simulink model "teppo"  (R2019a)
settings: Solver=VariableStepAuto  StartTime=0.0  StopTime=10.0  RelTol=1e-3
libraries: simulink x4, vrlib x2, visionsinks x1
settings Model: Creator=Arjun  LastModifiedBy=Arjun
settings DebuggingCC: UnderSpecifiedDimensionMsg=warning

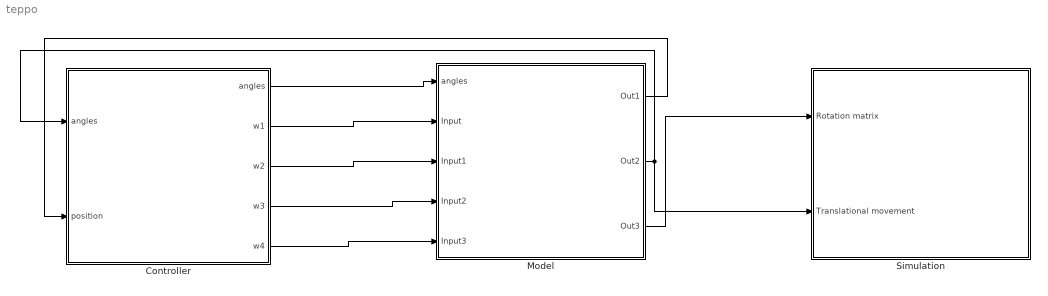
== system teppo ==
  "Controller " : Subsystem
  Model : Subsystem
  Simulation : Subsystem
  wires:
  "Controller "/1("angles ") -> Model/1("angles ")
  Model/3(Out3) -> Simulation/1(Rotation matrix)
  Model/1(Out1) -> "Controller "/2(position)
  Model/2(Out2) -> "Controller "/1(angles), Simulation/2(Translational movement)
  "Controller "/2(w1) -> Model/2(Input)
  "Controller "/3(w2) -> Model/3(Input1)
  "Controller "/4(w3) -> Model/4(Input2)
  "Controller "/5(w4) -> Model/5(Input3)

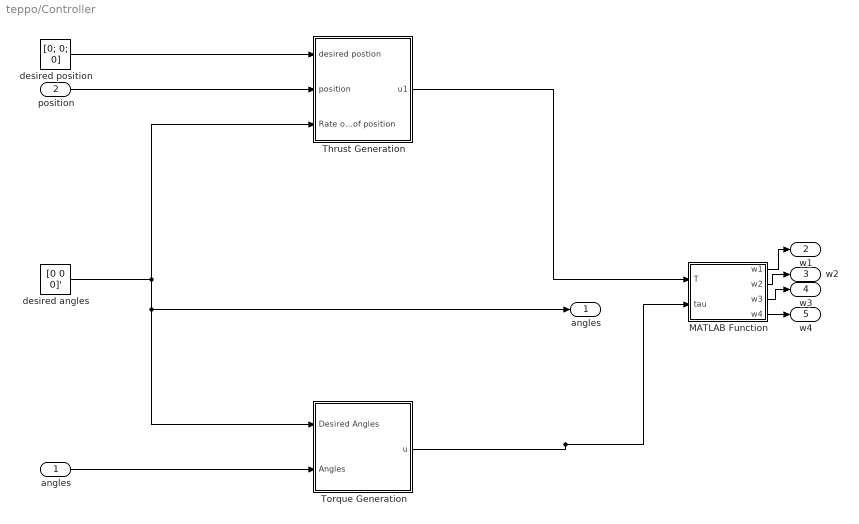
== system teppo/Controller  ==
  angles : Inport
  position : Inport  Port=2
  MATLAB Function : MATLAB Function  TreatAsAtomicUnit=on
  Thrust Generation : Subsystem
  Torque Generation : Subsystem
  desired angles : Constant  Value=[0 0 0]'
  desired position : Constant  Value=[0; 0; 0]
  "angles " : Outport
  w1 : Outport  Port=2
  w2 : Outport  Port=3
  w3 : Outport  Port=4
  w4 : Outport  Port=5
  wires:
  desired angles/1 -> Torque Generation/1("Desired Angles "), "angles "/1, Thrust Generation/3("Rate of change of position ")
  desired position/1 -> Thrust Generation/1("desired postion ")
  position/1 -> Thrust Generation/2(position)
  Thrust Generation/1(u1) -> MATLAB Function/1(T)
  angles/1 -> Torque Generation/2(Angles)
  Torque Generation/1(u) -> MATLAB Function/2(tau)
  MATLAB Function/1(w1) -> w1/1
  MATLAB Function/2(w2) -> w2/1
  MATLAB Function/3(w3) -> w3/1
  MATLAB Function/4(w4) -> w4/1

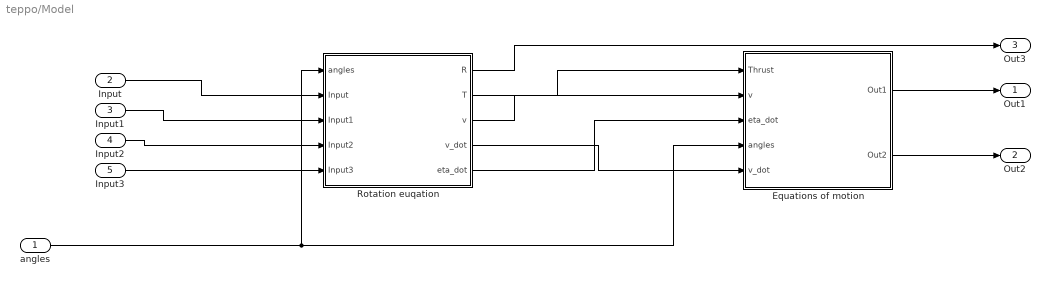
== system teppo/Model ==
  "angles " : Inport
  Input : Inport  Port=2
  Input1 : Inport  Port=3
  Input2 : Inport  Port=4
  Input3 : Inport  Port=5
  Equations of motion : Subsystem
  Rotation euqation : Subsystem
  Out1 : Outport
  Out2 : Outport  Port=2
  Out3 : Outport  Port=3
  wires:
  Rotation euqation/2(T) -> Equations of motion/1(Thrust)
  Rotation euqation/3("v ") -> Equations of motion/2("v ")
  "angles "/1 -> Equations of motion/4("angles "), Rotation euqation/1(angles)
  Rotation euqation/4("v_dot ") -> Equations of motion/5(v_dot)
  Equations of motion/2(Out2) -> Out2/1
  Equations of motion/1(Out1) -> Out1/1
  Rotation euqation/1(R) -> Out3/1
  Input/1 -> Rotation euqation/2(Input)
  Input1/1 -> Rotation euqation/3(Input1)
  Input2/1 -> Rotation euqation/4(Input2)
  Input3/1 -> Rotation euqation/5(Input3)
  Rotation euqation/5(eta_dot) -> Equations of motion/3("eta_dot ")

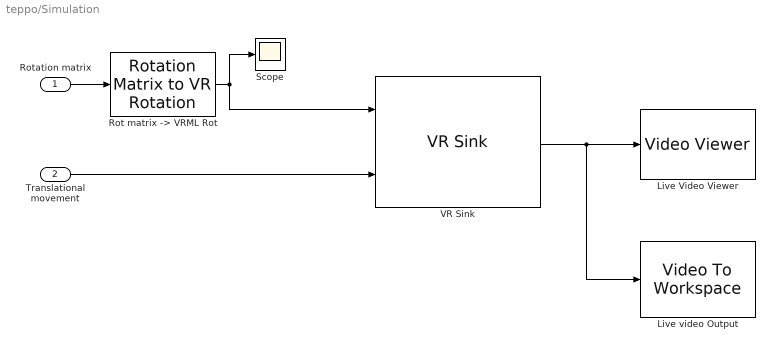
== system teppo/Simulation ==
  Rotation matrix : Inport
  Translational movement : Inport  Port=2
  Live Video Viewer : VideoViewer  FigPos=[1287 1075 375 346]
  Live video Output : visionsinks/Video To Workspace  VariableName=output  NumInputs=1  DataLimit=10  DecimationFactor=1  LogFi=off  InPortLabels=R|G|B
      settings: SourceProductName=Computer Vision Toolbox  SourceProductBaseCode=VP
  "Rot matrix -> VRML Rot" : vrlib/Utilities/Rotation Matrix to VR Rotation  maxzero=0
      settings: SourceProductName=Simulink 3D Animation  SourceProductBaseCode=VR
  Scope : Scope
  VR Sink : vrlib/VR Sink  InstantiateOnLoad=on  SampleTime=0.1  ViewEnable=on  RemoteChange=off  RemoteView=off  FieldsWritten=Quadcopter.rotation.4.1.1.double#Quadcopter.translation.3.1.1.double  WorldFileName=Quadcopter.wrl  AutoView=off  VideoDimensions=[277 277]  AllowVariableSize=off
      settings: SourceProductName=Simulink
  wires:
  "Rot matrix -> VRML Rot"/1 -> VR Sink/1, Scope/1
  Rotation matrix/1 -> "Rot matrix -> VRML Rot"/1
  VR Sink/1 -> Live video Output/1, Live Video Viewer/1
  Translational movement/1 -> VR Sink/2

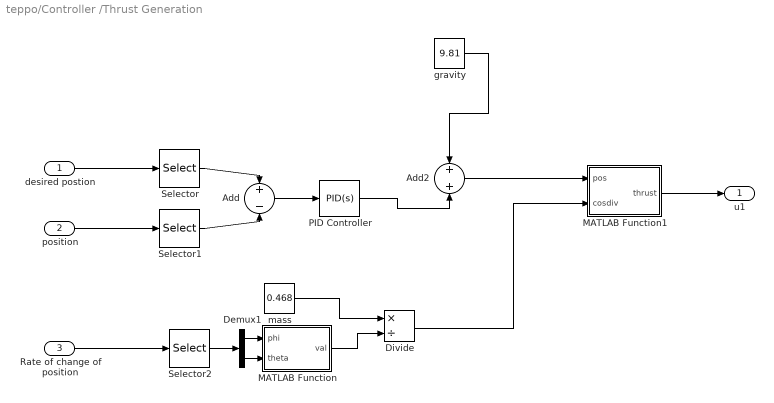
== system teppo/Controller /Thrust Generation ==
  "desired postion " : Inport
  position : Inport  Port=2
  "Rate of change of position " : Inport  Port=3
  Add : Sum  Inputs=+-
  Add2 : Sum
  Demux1 : Demux  Outputs=2
  Divide : Product  Inputs=*/
  MATLAB Function : MATLAB Function  TreatAsAtomicUnit=on
  MATLAB Function1 : MATLAB Function  TreatAsAtomicUnit=on
  PID Controller : simulink/Continuous/PID Controller  Controller=PID  Form=Parallel  TimeDomain=Continuous-time  SampleTime=-1  IntegratorMethod=Forward Euler  FilterMethod=Forward Euler  ControllerParametersSource=internal  P=1.5  I=1  D=2.5  UseFilter=on  N=100  TunerSelectOption=Transfer Function Based (PID Tuner App)  InitialConditionSource=internal  InitialConditionForIntegrator=0  InitialConditionForFilter=0  DifferentiatorICPrevScaledInput=0  ExternalReset=none  TrackingMode=off  Kt=1  LimitOutput=off  UpperSaturationLimit=inf  LowerSaturationLimit=-inf  LinearizeAsGain=on  AntiWindupMode=none  Kb=1  POutMin=[]  POutMax=[]  IOutMin=[]  IOutMax=[]  DOutMin=[]  DOutMax=[]  NOutMin=[]  NOutMax=[]  SumOutMin=[]  SumOutMax=[]  SaturationOutMin=[]  SaturationOutMax=[]  PParamMin=[]  PParamMax=[]  IParamMin=[]  IParamMax=[]  DParamMin=[]  DParamMax=[]  NParamMin=[]  NParamMax=[]  KbParamMin=[]  KbParamMax=[]  KtParamMin=[]  KtParamMax=[]  KbOutMin=[]  KbOutMax=[]  KtOutMin=[]  KtOutMax=[]  IntegratorOutMin=[]  IntegratorOutMax=[]  FilterOutMin=[]  FilterOutMax=[]  SumI1OutMin=[]  SumI1OutMax=[]  SumI2OutMin=[]  SumI2OutMax=[]  SumI3OutMin=[]  SumI3OutMax=[]  SumI4OutMin=[]  SumI4OutMax=[]  SumDOutMin=[]  SumDOutMax=[]  DifferentiatorOutMin=[]  DifferentiatorOutMax=[]  FilterDiffOutCoefMin=[]  FilterDiffOutCoefMax=[]  ReciprocalOutMin=[]  ReciprocalOutMax=[]  SumDenOutMin=[]  SumDenOutMax=[]  SumNumOutMin=[]  SumNumOutMax=[]  DivideOutMin=[]  DivideOutMax=[]  IntegratorContinuousStateAttributes=''  IntegratorStateMustResolveToSignalObject=off  IntegratorRTWStateStorageClass=Auto  FilterContinuousStateAttributes=''  FilterStateMustResolveToSignalObject=off  FilterRTWStateStorageClass=Auto  ParallelPVariant=InternalParameters  IdealPVariant=Disabled  IVariant=InternalParameters  DVariant=InternalParameters  IntegratorVariant=Continuous  SatVariant=Disabled  AWVariant=Passthrough  PCopyVariant=Disabled  TRVariant=Disabled  FdbkBlocksVariant=Forward  IdealPFdbkVariant=Disabled  SatFdbkVariant=Disabled  DerivativeFilterVariant=ContFilter  NVariant=InternalParameters  NCopyVariant=Disabled  FilterICVariant=InternalICsFilter  IntegratorICVariant=InternalICs  ExternalResetVariant=Disabled  TRSumVariant=Passthrough  SumFdbkVariant=Disabled  SumVariant=Sum_PID
  Selector : Selector  InputPortWidth=3  IndexOptions=Index vector (dialog)  Indices=[3]  OutputSizes=1
  Selector1 : Selector  InputPortWidth=3  IndexOptions=Index vector (dialog)  Indices=[3]  OutputSizes=1
  Selector2 : Selector  InputPortWidth=3  IndexOptions=Index vector (dialog)  Indices=[1 2]  OutputSizes=1
  "gravity " : Constant  Value=9.81
  "mass " : Constant  Value=0.468
  u1 : Outport
  wires:
  "mass "/1 -> Divide/1
  "desired postion "/1 -> Selector/1
  Demux1/2 -> MATLAB Function/2(theta)
  Demux1/1 -> MATLAB Function/1(phi)
  Divide/1 -> MATLAB Function1/2(cosdiv)
  Add2/1 -> MATLAB Function1/1(pos)
  MATLAB Function/1(val) -> Divide/2
  Selector2/1 -> Demux1/1
  MATLAB Function1/1(thrust) -> u1/1
  "Rate of change of position "/1 -> Selector2/1
  "gravity "/1 -> Add2/1
  position/1 -> Selector1/1
  Selector/1 -> Add/1
  Selector1/1 -> Add/2
  Add/1 -> PID Controller/1
  PID Controller/1 -> Add2/2

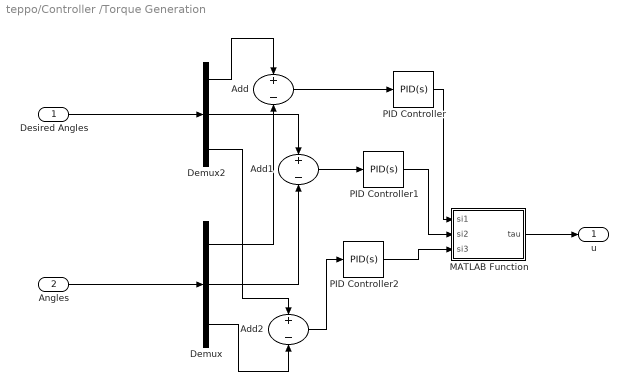
== system teppo/Controller /Torque Generation ==
  "Desired Angles " : Inport
  Angles : Inport  Port=2
  Add : Sum  Inputs=+-
  Add1 : Sum  Inputs=+-
  Add2 : Sum  Inputs=+-
  Demux : Demux  Outputs=3
  Demux2 : Demux  Outputs=3
  MATLAB Function : MATLAB Function  TreatAsAtomicUnit=on
  PID Controller : simulink/Continuous/PID Controller  Controller=PID  Form=Parallel  TimeDomain=Continuous-time  SampleTime=-1  IntegratorMethod=Forward Euler  FilterMethod=Forward Euler  ControllerParametersSource=internal  P=1  I=1  D=0  UseFilter=on  N=100  TunerSelectOption=Transfer Function Based (PID Tuner App)  InitialConditionSource=internal  InitialConditionForIntegrator=0  InitialConditionForFilter=0  DifferentiatorICPrevScaledInput=0  ExternalReset=none  TrackingMode=off  Kt=1  LimitOutput=off  UpperSaturationLimit=inf  LowerSaturationLimit=-inf  LinearizeAsGain=on  AntiWindupMode=none  Kb=1  POutMin=[]  POutMax=[]  IOutMin=[]  IOutMax=[]  DOutMin=[]  DOutMax=[]  NOutMin=[]  NOutMax=[]  SumOutMin=[]  SumOutMax=[]  SaturationOutMin=[]  SaturationOutMax=[]  PParamMin=[]  PParamMax=[]  IParamMin=[]  IParamMax=[]  DParamMin=[]  DParamMax=[]  NParamMin=[]  NParamMax=[]  KbParamMin=[]  KbParamMax=[]  KtParamMin=[]  KtParamMax=[]  KbOutMin=[]  KbOutMax=[]  KtOutMin=[]  KtOutMax=[]  IntegratorOutMin=[]  IntegratorOutMax=[]  FilterOutMin=[]  FilterOutMax=[]  SumI1OutMin=[]  SumI1OutMax=[]  SumI2OutMin=[]  SumI2OutMax=[]  SumI3OutMin=[]  SumI3OutMax=[]  SumI4OutMin=[]  SumI4OutMax=[]  SumDOutMin=[]  SumDOutMax=[]  DifferentiatorOutMin=[]  DifferentiatorOutMax=[]  FilterDiffOutCoefMin=[]  FilterDiffOutCoefMax=[]  ReciprocalOutMin=[]  ReciprocalOutMax=[]  SumDenOutMin=[]  SumDenOutMax=[]  SumNumOutMin=[]  SumNumOutMax=[]  DivideOutMin=[]  DivideOutMax=[]  IntegratorContinuousStateAttributes=''  IntegratorStateMustResolveToSignalObject=off  IntegratorRTWStateStorageClass=Auto  FilterContinuousStateAttributes=''  FilterStateMustResolveToSignalObject=off  FilterRTWStateStorageClass=Auto  ParallelPVariant=InternalParameters  IdealPVariant=Disabled  IVariant=InternalParameters  DVariant=InternalParameters  IntegratorVariant=Continuous  SatVariant=Disabled  AWVariant=Passthrough  PCopyVariant=Disabled  TRVariant=Disabled  FdbkBlocksVariant=Forward  IdealPFdbkVariant=Disabled  SatFdbkVariant=Disabled  DerivativeFilterVariant=ContFilter  NVariant=InternalParameters  NCopyVariant=Disabled  FilterICVariant=InternalICsFilter  IntegratorICVariant=InternalICs  ExternalResetVariant=Disabled  TRSumVariant=Passthrough  SumFdbkVariant=Disabled  SumVariant=Sum_PID
  PID Controller1 : simulink/Continuous/PID Controller  Controller=PID  Form=Parallel  TimeDomain=Continuous-time  SampleTime=-1  IntegratorMethod=Forward Euler  FilterMethod=Forward Euler  ControllerParametersSource=internal  P=1  I=1  D=0  UseFilter=on  N=100  TunerSelectOption=Transfer Function Based (PID Tuner App)  InitialConditionSource=internal  InitialConditionForIntegrator=0  InitialConditionForFilter=0  DifferentiatorICPrevScaledInput=0  ExternalReset=none  TrackingMode=off  Kt=1  LimitOutput=off  UpperSaturationLimit=inf  LowerSaturationLimit=-inf  LinearizeAsGain=on  AntiWindupMode=none  Kb=1  POutMin=[]  POutMax=[]  IOutMin=[]  IOutMax=[]  DOutMin=[]  DOutMax=[]  NOutMin=[]  NOutMax=[]  SumOutMin=[]  SumOutMax=[]  SaturationOutMin=[]  SaturationOutMax=[]  PParamMin=[]  PParamMax=[]  IParamMin=[]  IParamMax=[]  DParamMin=[]  DParamMax=[]  NParamMin=[]  NParamMax=[]  KbParamMin=[]  KbParamMax=[]  KtParamMin=[]  KtParamMax=[]  KbOutMin=[]  KbOutMax=[]  KtOutMin=[]  KtOutMax=[]  IntegratorOutMin=[]  IntegratorOutMax=[]  FilterOutMin=[]  FilterOutMax=[]  SumI1OutMin=[]  SumI1OutMax=[]  SumI2OutMin=[]  SumI2OutMax=[]  SumI3OutMin=[]  SumI3OutMax=[]  SumI4OutMin=[]  SumI4OutMax=[]  SumDOutMin=[]  SumDOutMax=[]  DifferentiatorOutMin=[]  DifferentiatorOutMax=[]  FilterDiffOutCoefMin=[]  FilterDiffOutCoefMax=[]  ReciprocalOutMin=[]  ReciprocalOutMax=[]  SumDenOutMin=[]  SumDenOutMax=[]  SumNumOutMin=[]  SumNumOutMax=[]  DivideOutMin=[]  DivideOutMax=[]  IntegratorContinuousStateAttributes=''  IntegratorStateMustResolveToSignalObject=off  IntegratorRTWStateStorageClass=Auto  FilterContinuousStateAttributes=''  FilterStateMustResolveToSignalObject=off  FilterRTWStateStorageClass=Auto  ParallelPVariant=InternalParameters  IdealPVariant=Disabled  IVariant=InternalParameters  DVariant=InternalParameters  IntegratorVariant=Continuous  SatVariant=Disabled  AWVariant=Passthrough  PCopyVariant=Disabled  TRVariant=Disabled  FdbkBlocksVariant=Forward  IdealPFdbkVariant=Disabled  SatFdbkVariant=Disabled  DerivativeFilterVariant=ContFilter  NVariant=InternalParameters  NCopyVariant=Disabled  FilterICVariant=InternalICsFilter  IntegratorICVariant=InternalICs  ExternalResetVariant=Disabled  TRSumVariant=Passthrough  SumFdbkVariant=Disabled  SumVariant=Sum_PID
  PID Controller2 : simulink/Continuous/PID Controller  Controller=PID  Form=Parallel  TimeDomain=Continuous-time  SampleTime=-1  IntegratorMethod=Forward Euler  FilterMethod=Forward Euler  ControllerParametersSource=internal  P=1  I=1  D=0  UseFilter=on  N=100  TunerSelectOption=Transfer Function Based (PID Tuner App)  InitialConditionSource=internal  InitialConditionForIntegrator=0  InitialConditionForFilter=0  DifferentiatorICPrevScaledInput=0  ExternalReset=none  TrackingMode=off  Kt=1  LimitOutput=off  UpperSaturationLimit=inf  LowerSaturationLimit=-inf  LinearizeAsGain=on  AntiWindupMode=none  Kb=1  POutMin=[]  POutMax=[]  IOutMin=[]  IOutMax=[]  DOutMin=[]  DOutMax=[]  NOutMin=[]  NOutMax=[]  SumOutMin=[]  SumOutMax=[]  SaturationOutMin=[]  SaturationOutMax=[]  PParamMin=[]  PParamMax=[]  IParamMin=[]  IParamMax=[]  DParamMin=[]  DParamMax=[]  NParamMin=[]  NParamMax=[]  KbParamMin=[]  KbParamMax=[]  KtParamMin=[]  KtParamMax=[]  KbOutMin=[]  KbOutMax=[]  KtOutMin=[]  KtOutMax=[]  IntegratorOutMin=[]  IntegratorOutMax=[]  FilterOutMin=[]  FilterOutMax=[]  SumI1OutMin=[]  SumI1OutMax=[]  SumI2OutMin=[]  SumI2OutMax=[]  SumI3OutMin=[]  SumI3OutMax=[]  SumI4OutMin=[]  SumI4OutMax=[]  SumDOutMin=[]  SumDOutMax=[]  DifferentiatorOutMin=[]  DifferentiatorOutMax=[]  FilterDiffOutCoefMin=[]  FilterDiffOutCoefMax=[]  ReciprocalOutMin=[]  ReciprocalOutMax=[]  SumDenOutMin=[]  SumDenOutMax=[]  SumNumOutMin=[]  SumNumOutMax=[]  DivideOutMin=[]  DivideOutMax=[]  IntegratorContinuousStateAttributes=''  IntegratorStateMustResolveToSignalObject=off  IntegratorRTWStateStorageClass=Auto  FilterContinuousStateAttributes=''  FilterStateMustResolveToSignalObject=off  FilterRTWStateStorageClass=Auto  ParallelPVariant=InternalParameters  IdealPVariant=Disabled  IVariant=InternalParameters  DVariant=InternalParameters  IntegratorVariant=Continuous  SatVariant=Disabled  AWVariant=Passthrough  PCopyVariant=Disabled  TRVariant=Disabled  FdbkBlocksVariant=Forward  IdealPFdbkVariant=Disabled  SatFdbkVariant=Disabled  DerivativeFilterVariant=ContFilter  NVariant=InternalParameters  NCopyVariant=Disabled  FilterICVariant=InternalICsFilter  IntegratorICVariant=InternalICs  ExternalResetVariant=Disabled  TRSumVariant=Passthrough  SumFdbkVariant=Disabled  SumVariant=Sum_PID
  u : Outport
  wires:
  "Desired Angles "/1 -> Demux2/1
  Angles/1 -> Demux/1
  MATLAB Function/1(tau) -> u/1
  Demux2/1 -> Add/1
  Demux/1 -> Add/2
  Add/1 -> PID Controller/1
  Demux2/2 -> Add1/1
  Demux/2 -> Add1/2
  Add1/1 -> PID Controller1/1
  Demux2/3 -> Add2/1
  Demux/3 -> Add2/2
  Add2/1 -> PID Controller2/1
  PID Controller2/1 -> MATLAB Function/3(si3)
  PID Controller1/1 -> MATLAB Function/2(si2)
  PID Controller/1 -> MATLAB Function/1(si1)

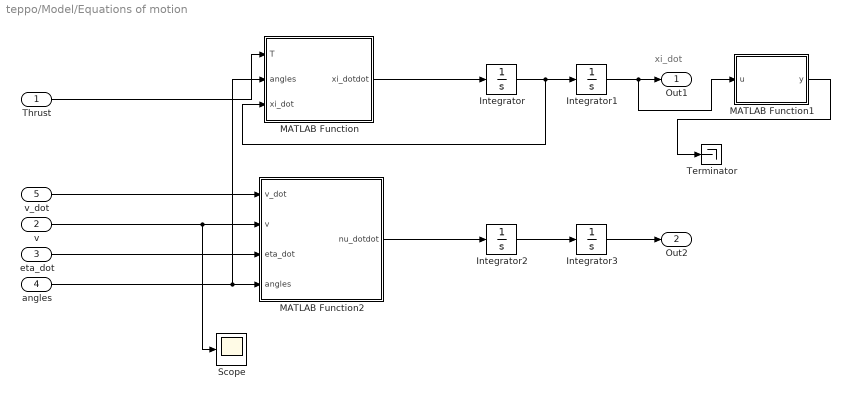
== system teppo/Model/Equations of motion ==
  note: xi_dot
  Thrust : Inport
  "v " : Inport  Port=2
  "eta_dot " : Inport  Port=3
  "angles " : Inport  Port=4
  v_dot : Inport  Port=5
  Integrator{,1..3} (4 alike) : Integrator
  MATLAB Function : MATLAB Function  TreatAsAtomicUnit=on
  MATLAB Function1 : MATLAB Function  TreatAsAtomicUnit=on
  MATLAB Function2 : MATLAB Function  TreatAsAtomicUnit=on
  Scope : Scope
  Terminator : Terminator
  Out1 : Outport
  Out2 : Outport  Port=2
  wires:
  MATLAB Function/1(xi_dotdot) -> Integrator/1
  v_dot/1 -> MATLAB Function2/1(v_dot)
  "eta_dot "/1 -> MATLAB Function2/3(eta_dot)
  "v "/1 -> Scope/1, MATLAB Function2/2(v)
  "angles "/1 -> MATLAB Function/2(angles), MATLAB Function2/4(angles)
  Thrust/1 -> MATLAB Function/1(T)
  Integrator/1 -> MATLAB Function/3(xi_dot), Integrator1/1
  Integrator1/1 -> MATLAB Function1/1(u), Out1/1
  MATLAB Function2/1(nu_dotdot) -> Integrator2/1
  Integrator3/1 -> Out2/1
  Integrator2/1 -> Integrator3/1
  MATLAB Function1/1(y) -> Terminator/1

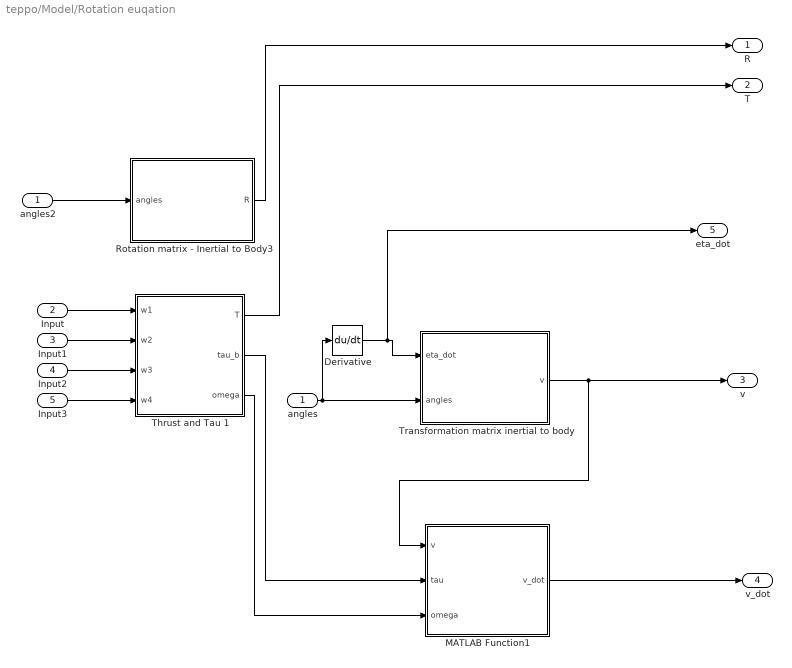
== system teppo/Model/Rotation euqation ==
  angles : Inport
  Input : Inport  Port=2
  Input1 : Inport  Port=3
  Input2 : Inport  Port=4
  Input3 : Inport  Port=5
  Derivative : Derivative
  MATLAB Function1 : MATLAB Function  TreatAsAtomicUnit=on
  Rotation matrix - Inertial to Body3 : MATLAB Function  TreatAsAtomicUnit=on
  Thrust and Tau 1 : MATLAB Function  TreatAsAtomicUnit=on
  Transformation matrix inertial to body : MATLAB Function  TreatAsAtomicUnit=on
  angles2 : InportShadow
  R : Outport
  T : Outport  Port=2
  "v " : Outport  Port=3
  "v_dot " : Outport  Port=4
  eta_dot : Outport  Port=5
  wires:
  Transformation matrix inertial to body/1(v) -> MATLAB Function1/1(v), "v "/1
  angles/1 -> Transformation matrix inertial to body/2(angles), Derivative/1
  Thrust and Tau 1/1(T) -> T/1
  Rotation matrix - Inertial to Body3/1(R) -> R/1
  MATLAB Function1/1(v_dot) -> "v_dot "/1
  angles2/1 -> Rotation matrix - Inertial to Body3/1(angles)
  Input/1 -> Thrust and Tau 1/1(w1)
  Input1/1 -> Thrust and Tau 1/2(w2)
  Input2/1 -> Thrust and Tau 1/3(w3)
  Input3/1 -> Thrust and Tau 1/4(w4)
  Derivative/1 -> eta_dot/1, Transformation matrix inertial to body/1(eta_dot)
  Thrust and Tau 1/2(tau_b) -> MATLAB Function1/2(tau)
  Thrust and Tau 1/3(omega) -> MATLAB Function1/3(omega)

== matlab function teppo/Controller /Thrust Generation/MATLAB Function1 ==
  data: pos input; thrust output; cosdiv input
function thrust = fcn(pos, cosdiv)
    thrust = pos * cosdiv;

== matlab function teppo/Controller /Thrust Generation/MATLAB Function ==
  data: phi input; val output; theta input
function val = fcn(phi, theta)
    val = cos(phi) * cos(theta);

== matlab function teppo/Controller /Torque Generation/MATLAB Function ==
  data: si1 input; tau output; si2 input; si3 input
function tau = fcn(si1, si2, si3)
    tau = [si1; si2; si3];

== matlab function teppo/Controller /MATLAB Function ==
  data: w1 output; T input; tau input; w2 output; w3 output; w4 output
function [w1,w2,w3,w4] = fcn(T, tau)
    k = 2.980 * 10 ^-6; % 2.9800e-06 lift constant
    b = 1.140 * 10 ^-7;   % 1.1400e-07 drag constant
    l = 0.225; % distance between rotors    
    
    w1 = (T/4*k)-(tau(2)/2*k*l)-(tau(3)/4*b);
    w2 = (T/4*k)-(tau(1)/2*k*l)-(tau(3)/4*b);
    w3 = (T/4*k)+(tau(2)/2*k*l)-(tau(3)/4*b);
    w4 = (T/4*k)+(tau(1)/2*k*l)+(tau(3)/4*b);

== matlab function teppo/Model/Equations of motion/MATLAB Function1 ==
  data: u input; y output
function y = fcn(u)
Simulatoras.Simulator();
y = u;

== matlab function teppo/Model/Rotation euqation/Rotation matrix - Inertial to Body3 ==
  data: angles input; R output
function R = fcn(angles)
    
    phi = angles(1);
    theta = angles(2);
    psi = angles(3);
    
    R = [cos(psi) * cos(theta) cos(psi) * sin(theta) * sin(phi) - sin(psi) * cos(phi) cos(psi) * sin(theta) * cos(phi) + sin(psi) * sin(phi);
		  sin(psi) * cos(theta) sin(psi) * sin(theta) * sin(phi) + cos(psi) * cos(phi) sin(psi) * sin(theta) * cos(phi) - cos(psi) * sin(phi);
		  -sin(theta) cos(theta) * sin(phi) cos(theta) * cos(phi)]';

== matlab function teppo/Model/Rotation euqation/Thrust and Tau 1 ==
  data: w1 input; T output; tau_b output; w2 input; omega output; w3 input; w4 input
function [T, tau_b, omega] = fcn(w1, w2, w3, w4)

    k = 2.980 * 10 ^-6; % 2.9800e-06 lift constant
    b = 1.140 * 10 ^-7;   % 1.1400e-07 drag constant
    Im = 3.357 * 10 ^-5; % Inertia moment of rotors
    l = 0.225; % distance between rotors
    km = 2 * 10 ^-6;
    
    
    omega_1 = sqrt(abs(w1));
    omega_2 = sqrt(abs(w2));
    omega_3 = sqrt(abs(w3));
    omega_4 = sqrt(abs(w4));
    omega = [omega_1; omega_2; omega_3; omega_4];
    
    % f_i = kw_i ^ 2; force
    f1 = k * (w1);
    f2 = k * (w2);
    f3 = k * (w3);
    f4 = k * (w4);
    
    % tau_m_i = b * w_i ^ 2 + I_m => Torque of each propeller
    tau_m1 = b * (w1) + Im;
    tau_m2 = b * (w2) + Im;
    tau_m3 = b * (w3) + Im;
    tau_m4 = b * (w4) + Im;
%     torque = tau_m1 + tau_m2 + tau_m3 + tau_m4;
    
    % sigma(f_i) => T Thrust
    T = f1 + f2 + f3 + f4;
%     T_B = [0; 0; T]
    

    tau_phi = (l * k) * (-(w2) + (w4));
    tau_theta = (l * k) * (-(w1) + (w3));
    tau_psi = tau_m1 + tau_m2 + tau_m3 + tau_m4;
         
    tau_b = [tau_phi tau_theta tau_psi]';

== matlab function teppo/Model/Rotation euqation/Transformation matrix inertial to body ==
  data: eta_dot input; v output; angles input
function v = fcn(eta_dot,angles)
%     phi_dot = eta_dot(1);
%     theta_dot = eta_dot(2);
%     psi_dot = eta_dot(3);
    phi = angles(1);
    theta = angles(2);
    W_eta = [1 0 -sin(phi);
            0 cos(phi) cos(theta) * sin(phi); 
            0 -sin(phi) cos(theta) * cos(phi)
    ];
    
    v = W_eta * eta_dot;

== matlab function teppo/Model/Equations of motion/MATLAB Function ==
  data: xi_dotdot output; T input; angles input; xi_dot input
function xi_dotdot = fcn(T, angles, xi_dot)
   phi = angles(1);
   theta = angles(2);
   psi = angles(3);
   g = 9.81;
   m = 0.468;
   R = [cos(psi) * sin(theta)*cos(phi) + sin(psi) * sin(phi);
        sin(psi)*sin(theta)*cos(phi) - cos(psi)*sin(phi);
        cos(theta)*cos(phi)
   ];
    Ax = 0.25;
    Ay = 0.25; 
    Az = 0.25;
    xi_dotdot = [0 0 -g]' + (T/m) * R;  % getting error here
    % Aerodynamic effects
    
    xi_dotdot = xi_dotdot - 1/m * [Ax 0 0; 0 Ay 0; 0 0 Az] * [x_dot y_dot z_dot];

== matlab function teppo/Model/Rotation euqation/MATLAB Function1 ==
  data: v input; v_dot output; tau input; omega input
function v_dot = fcn(v, tau, omega)
%     Ixx = 0.0049;
%     Iyy = 0.0049;
%     Izz = 0.0088;
%     omega_1 = omega(1);
%     omega_2 = omega(2);
%     omega_3 = omega(3);
%     omega_4 = omega(4);
%     
%     I = diag([Ixx, Iyy, Izz]);
%     omega_gamma = omega_1 - omega_2 + omega_3 - omega_4;
% %     v_dot = I \ ();
v_dot = [10, 20, 30]';

%     v_dot = inv(I) * cross(-v, [Ixx * p; Iyy * q; Izz * r]) - I * cross(v, [0; 0; 1]) * omega_gamma + tau

%     v_dot = [0 0 0]';
    
    %v_dot = tau - v * IV - omega_gamma;

== matlab function teppo/Model/Equations of motion/MATLAB Function2 ==
  data: v_dot input; nu_dotdot output; v input; eta_dot input; angles input
function nu_dotdot = fcn(v_dot, v, eta_dot, angles)
    
    phi_dot = eta_dot(1);
    theta_dot = eta_dot(2);
    psi_dot = eta_dot(3);
    phi = angles(1);
    theta = angles(2);
    psi = angles(3);
    W_n = [1 sin(phi)*tan(theta) cos(phi)*tan(theta);
           0 cos(phi) -sin(phi);
           0 sin(phi)/cos(theta) cos(phi)/cos(theta)
        ];
    nu_dotdot = [0 phi_dot * cos(phi) * tan(theta) + theta_dot * sin(phi)/cos(theta)^2 -phi_dot * sin(phi) * cos(theta) + theta_dot * cos(phi)/cos(theta) ^ 2;
     0 -phi_dot * sin(phi) -phi_dot * cos(phi);
     0 phi_dot * cos(phi) / cos(theta) +phi_dot * sin(phi) * tan(theta) / cos(theta) -phi_dot * sin(phi)/cos(theta) + theta_dot * cos(phi) * tan(theta)/cos(theta)
     ] * v + W_n * v_dot;
